simulink model "finalsimple_VER"  (R2023b)
settings: Solver=VariableStepAuto  StartTime=0.0  StopTime=5  FixedStep=4  MaxStep=0.01  RelTol=1e-3
undefined symbols (not defined in the file or in its folder): Ion, Lithium
libraries: simulink x40, nesl_utility x10, spsSeriesRLCBranchLib x8, fl_lib x6, spsMosfetLib x6, dspsrcs4 x5, spsControlledCurrentSourceLib x5, ee_lib x4, spsCurrentMeasurementLib x4, spsVoltageMeasurementLib x4, spsBatteryLib x3, spsGroundLib x2
(part 1 of 2)
settings Model: Creator=yeowy  LastModifiedBy=yeowy
settings DataIOCC: SaveFinalState=on  SaveOperatingPoint=on  SaveFormat=StructureWithTime

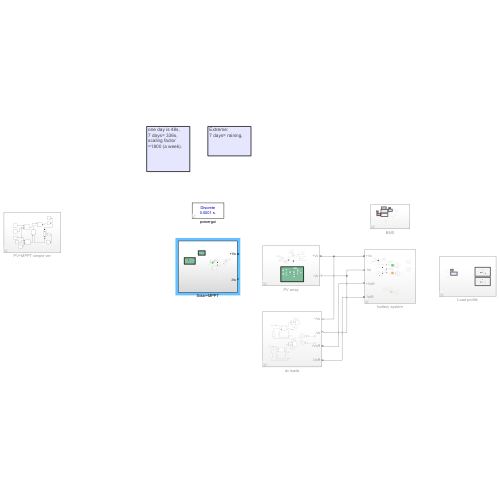
[thumbnail: Simulink's stored preview of the top-level diagram]
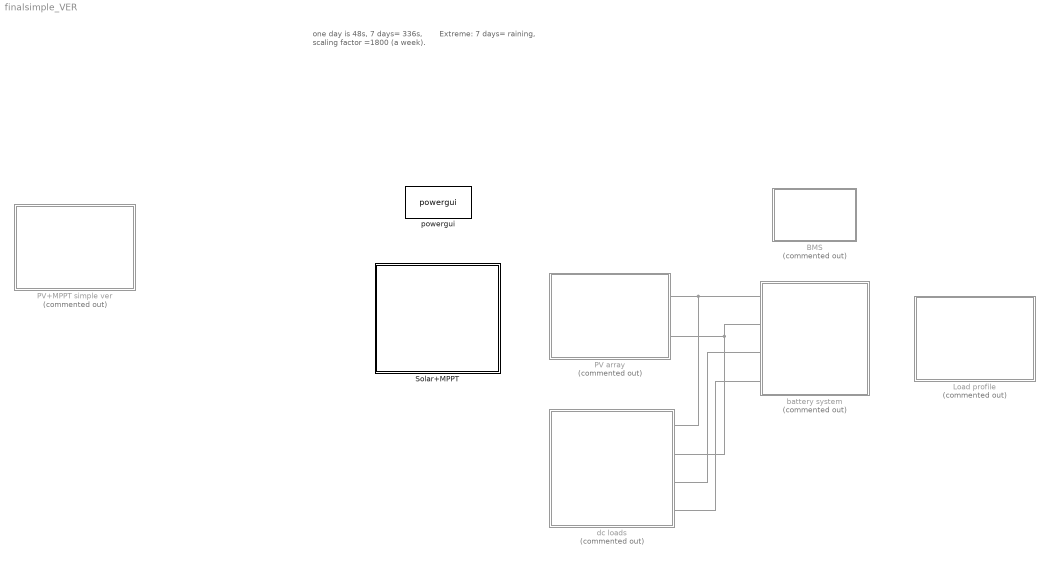
== system finalsimple_VER ==
  note: Extreme:
      | 7 days= raining,
  note: one day is 48s,
      | 7 days= 336s,
      | scaling factor
      | =1800 (a week).
  BMS : Subsystem  Commented=on
  Load profile : Subsystem  Commented=on
  PV array : Subsystem  Commented=on
  PV+MPPT simple ver : Subsystem  Commented=on
  Solar+MPPT : Subsystem
  battery system : Subsystem  Commented=on
  dc loads : Subsystem  Commented=on
  powergui : sps_lib/powergui  Priority=1  SimulationMode=Discrete  SampleTime=1e-4  frequency=60  Iterations=50  frequencyindice=0  Pbase=100e6  ErrMax=1e-4  UnitsV=kV  UnitsW=MW  buscounter=0  FunctionMessages=off  echomessages=off  EnableUseOfTLC=off  CurrentSourceSwitches=off  DisableSnubberDevices=off  DisableRonSwitches=off  DisableVfSwitches=off  DisplayEquations=off  AutomaticDiscreteSolvers=off  SolverType=Tustin/Backward Euler (TBE)  Interpol=off  ExternalGateDelay=off  methode=off  Ts=100  x0status=blocks  SPID=on  SwTol=0  HookPort=off  NonlinearTolerance=1e-4  nMaxIteration=100  ContinueOnMaxIteration=off  RestoreLinks=warning  ResistiveCurrentMeasurement=off  Frange=[0:2:500]  Ylog=off  Xlog=on  ShowGrid=off  save=off  variable=ZData  structure=0  ZoomFFT=off  StartTime=0.0  cycles=1  DisplayStyle=1  fundamental=60  FreqAxis=off  MaxFrequency=1000  frequencyindicesteady=1  RmsSteady=1  display=off
  connections:
  PV array/RConn1 -- dc loads/RConn1 -- battery system/LConn1
  battery system/LConn2 -- dc loads/RConn2 -- PV array/RConn2
  battery system/LConn3 -- dc loads/RConn3
  battery system/LConn4 -- dc loads/RConn4

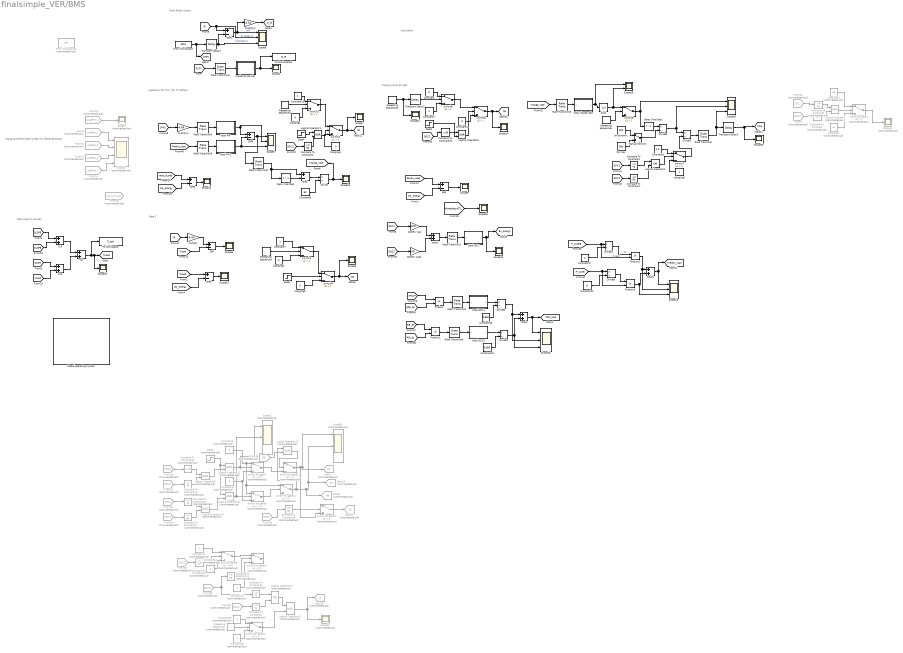
== system finalsimple_VER/BMS ==
  note: charging rover at night
  note: Calculation
  note: Total Load (in one day)
  note: Charging scheme:
      | 6pm to 6am for diesel generator
  note: Solar Panel system
  note: prediction (for tmr) (for PV battery)
  note: Gate 2
  Abs1 : Abs  SaturateOnIntegerOverflow=off
  Compare To Constant : simulink/Logic and Bit Operations/Compare To Constant  Commented=on  relop=<=  const=70  OutDataTypeStr=boolean
  Compare To Constant1 : simulink/Logic and Bit Operations/Compare To Constant  Commented=on  relop=>=  const=50  OutDataTypeStr=boolean
  Compare To Constant10 : simulink/Logic and Bit Operations/Compare To Constant  relop=>  const=85  OutDataTypeStr=boolean
  Compare To Constant11 : simulink/Logic and Bit Operations/Compare To Constant  Commented=on  relop=<=  const=20  OutDataTypeStr=boolean
  Compare To Constant12 : simulink/Logic and Bit Operations/Compare To Constant  Commented=on  relop=>  const=20  OutDataTypeStr=boolean
  Compare To Constant13 : simulink/Logic and Bit Operations/Compare To Constant  Commented=on  relop=<=  const=80  OutDataTypeStr=boolean
  Compare To Constant14 : simulink/Logic and Bit Operations/Compare To Constant  Commented=on  relop=<=  const=85  OutDataTypeStr=boolean
  Compare To Constant15 : simulink/Logic and Bit Operations/Compare To Constant  Commented=on  relop=>=  const=70  OutDataTypeStr=boolean
  Compare To Constant16 : simulink/Logic and Bit Operations/Compare To Constant  Commented=on  relop=<=  const=20  OutDataTypeStr=boolean
  Compare To Constant17 : simulink/Logic and Bit Operations/Compare To Constant  Commented=on  relop=<=  const=80  OutDataTypeStr=boolean
  Compare To Constant18 : simulink/Logic and Bit Operations/Compare To Constant  Commented=on  relop===  const=80  OutDataTypeStr=boolean
  Compare To Constant2 : simulink/Logic and Bit Operations/Compare To Constant  relop=>=  const=90  OutDataTypeStr=boolean
  Compare To Constant3 : simulink/Logic and Bit Operations/Compare To Constant  relop=>=  const=70  OutDataTypeStr=boolean
  Compare To Constant4 : simulink/Logic and Bit Operations/Compare To Constant  relop=<=  const=50  OutDataTypeStr=boolean
  Compare To Constant9 : simulink/Logic and Bit Operations/Compare To Constant  Commented=on  relop=<=  const=20  OutDataTypeStr=boolean
  Constant : Constant  Value=0
  Constant1 : Constant
  Constant{4,11,14,19} (4 alike) : Constant  Commented=on
  Constant12 : Constant  Commented=on  Value=0
  Constant13 : Constant
  Constant15 : Constant  Value=9.950
  Constant16 : Constant  Value=9.950
  Constant17 : Constant  Value=4
  Constant18 : Constant  Commented=on  Value=0
  Constant2 : Constant  Value=0
  Constant20 : Constant  Value=6
  Constant3 : Constant  Commented=on  Value=0
  Constant5 : Constant  Commented=on  Value=40
  Constant6 : Constant  Value=50
  Constant7 : Constant
  Constant8 : Constant  Value=1.3
  Constant9 : Constant  Commented=on  Value=80
  Delay One Step : Delay  DelayLength=1
  Delay One Step1 : Delay  DelayLength=1  SampleTime=50
  Diesel operating system : Subsystem
  Diff{,1..5} (6 alike) : Sum  Inputs=+-
  Divide{,1..6} (7 alike) : Product  Inputs=*/  RndMeth=Zero  SaturateOnIntegerOverflow=on
  From Workspace : FromWorkspace  VariableName=data  SampleTime=50  OutputAfterFinalValue=Holding final value
  From Workspace1 : FromWorkspace  Commented=on  VariableName=PIR
  From10 : From  Commented=on  GotoTag=LoadPre_3  TagVisibility=global
  From12 : From  Commented=on  GotoTag=LoadPre_4  TagVisibility=global
  From13 : From  Commented=on  GotoTag=LoadPre_1  TagVisibility=global
  From14 : From  Commented=on  GotoTag=LoadPre_7  TagVisibility=global
  From20 : From  Commented=on  GotoTag=Next_2hLoad  TagVisibility=global
  From23 : From  Commented=on  GotoTag=SOC1  TagVisibility=global
  From30 : From  Commented=on  GotoTag=SOC3  TagVisibility=global
  From{7,32,35..37} (5 alike) : From  Commented=on  GotoTag=SOC2  TagVisibility=global
  From33 : From  Commented=on  GotoTag=SOC3  TagVisibility=global
  From34 : From  Commented=on  GotoTag=SOC3
  From38 : From  Commented=on  GotoTag=SOC3
  From39 : From  Commented=on  GotoTag=G5  TagVisibility=global
  From5 : From  Commented=on  GotoTag=LoadPre_2  TagVisibility=global
  Goto13 : Goto  Commented=on  GotoTag=L1  TagVisibility=global
  Goto14 : Goto  Commented=on  GotoTag=G4  TagVisibility=global
  Goto15 : Goto  Commented=on  GotoTag=G5  TagVisibility=global
  Goto7 : Goto  Commented=on  GotoTag=G2  TagVisibility=global
  Goto8 : Goto  Commented=on  GotoTag=G6  TagVisibility=global
  Logical Operator{,8,10..12,16} (6 alike) : Logic  Commented=on  AllPortsSameDT=off  OutDataTypeStr=boolean
  Logical Operator1 : Logic  Operator=XOR  AllPortsSameDT=off  OutDataTypeStr=boolean
  Logical Operator13 : Logic  Commented=on  Operator=XOR  AllPortsSameDT=off  OutDataTypeStr=boolean
  Logical Operator15 : Logic  Commented=on  Operator=OR  AllPortsSameDT=off  OutDataTypeStr=boolean
  Logical Operator2 : Logic  Operator=OR  AllPortsSameDT=off  OutDataTypeStr=boolean
  Logical Operator9 : Logic  Operator=XOR  AllPortsSameDT=off  OutDataTypeStr=boolean
  Manual Switch2 : ManualSwitch
  Multiply : Gain  Gain=4.64
  Multiply1 : Gain  Gain=4.64
  Multiply2 : Gain  Gain=4.64
  Product{,1..3} (4 alike) : Product
  Rate Transition : RateTransition  OutPortSampleTime=600
  Rate Transition1 : RateTransition  OutPortSampleTime=100
  Rate Transition{2..3,6,8..9} (5 alike) : RateTransition  OutPortSampleTime=50
  Rate Transition4 : RateTransition  OutPortSampleTime=100
  Rate Transition5 : RateTransition  OutPortSampleTime=100
  Repeating Sequence1 : simulink/Sources/Repeating Sequence  Commented=on  rep_seq_t=[0 300 300.1 900.99 901 1200]  rep_seq_y=[0.9 0.9 1.01 1.01 0.9 0.9]
  Repeating Sequence2 : simulink/Sources/Repeating Sequence  rep_seq_t=[0 300 300.1 900.99 901 1200]  rep_seq_y=[0.9 0.9 1.01 1.01 0.9 0.9]
  Repeating Sequence3 : simulink/Sources/Repeating Sequence  rep_seq_t=[0 300 300.1 900.99 901 1200]  rep_seq_y=[0.9 0.9 1.01 1.01 0.9 0.9]
  Repeating Sequence4 : simulink/Sources/Repeating Sequence  rep_seq_t=[0 300 300.1 900.99 901 1200]  rep_seq_y=[0.9 0.9 1.01 1.01 0.9 0.9]
  Repeating Sequence5 : simulink/Sources/Repeating Sequence  rep_seq_t=[0 1099.99 1100 1200 1200.1]  rep_seq_y=[0.9 0.9 1.01 1.01 0.9]
  Scope{1,4,7..10,12..15,17,23..25} (14 alike) : Scope
  Scope11 : Scope  Commented=on
  Scope{5..6,16,19,26} (5 alike) : Scope  NumInputPorts=3
  Scope18 : Scope  NumInputPorts=2
  Scope2 : Scope  Commented=on  NumInputPorts=4
  Scope20 : Scope  Commented=on  NumInputPorts=3
  Scope21 : Scope  Commented=on  NumInputPorts=3
  Scope22 : Scope  Commented=on
  Scope3 : Scope  Commented=on
  Step1 : Step  Time=2400  After=2  SampleTime=1
  Step2 : Step  Time=2400  After=2  SampleTime=1
  Step3 : Step  Commented=on  Time=2400  After=2  SampleTime=1
  Step4 : Step  Time=2400  After=2  SampleTime=1
  TL5 : Sum
  TL6 : Sum
  TL7 : Sum
  To Workspace : ToWorkspace  VariableName=TLoad  SampleTime=1
      settings: Decimation=2  Save2DSignal=2-D array (concatenate along first dimension)
  To Workspace1 : ToWorkspace  VariableName=D_IR  SampleTime=1
      settings: Decimation=2  Save2DSignal=2-D array (concatenate along first dimension)
  Transport Delay1 : TransportDelay  DelayTime=2400
  Transport Delay2 : TransportDelay  DelayTime=2400
  Transport Delay3 : TransportDelay  DelayTime=900
  battery cap : Gain  Gain=100
  battery cap1 : Gain  Gain=50
  charging{1..4} (4 alike) : Constant  Value=0
  charging5 : Constant
  for dynamic : Constant  Value=300
  for max : Constant  Value=500
  gap : Sum  Inputs=+-
  irradiance per day : MATLAB Function  TreatAsAtomicUnit=on
  switch for gate{1,11..13} (4 alike) : Switch  Commented=on  Criteria=u2 > Threshold  SaturateOnIntegerOverflow=off  InputSameDT=off
  switch for gate{7..10} (4 alike) : Switch  Commented=on  Criteria=u2 ~= 0  Threshold=1  SaturateOnIntegerOverflow=off  InputSameDT=off
  switch for gate14 : Switch  Commented=on  Criteria=u2 > Threshold  Threshold=1  SaturateOnIntegerOverflow=off  InputSameDT=off
  switch{1,3..6,8} (6 alike) : Switch  Criteria=u2 > Threshold  Threshold=1  SaturateOnIntegerOverflow=off  InputSameDT=off
  switch2 : Switch  Criteria=u2 > Threshold  SaturateOnIntegerOverflow=off  InputSameDT=off
  switch7 : Switch  Criteria=u2 > Threshold  SaturateOnIntegerOverflow=off  InputSameDT=off
  total PIR : MATLAB Function  TreatAsAtomicUnit=on
  total PIR1 : MATLAB Function  TreatAsAtomicUnit=on
  total SOC : MATLAB Function  TreatAsAtomicUnit=on
  total SOC1 : MATLAB Function  TreatAsAtomicUnit=on
  total SOC2 : MATLAB Function  TreatAsAtomicUnit=on
  total charge rate : MATLAB Function  TreatAsAtomicUnit=on
  total1 : Sum
  total2 : Sum
  total3 : Sum
  tag scope: Bs_energy=global, CR4=global, D_IR=global, G1=global, G2=global, G4=global, Predict_load=global, TDC_load=global, TLoad=global, charge_rate=global
  wires:
  Diff/1 -> Scope4/1
  From Workspace/1 -> [PIR], Transport Delay1/1
  Diff1/1 -> Multiply2/1, Scope6/1  "Diff"
  From14/1 -> Scope2/4
  From12/1 -> Scope2/3
  From10/1 -> Scope2/2
  From5/1 -> Scope2/1
  From13/1 -> Scope3/1
  [IR] -> Multiply/1
  Multiply/1 -> Diff/1
  Multiply1/1 -> Rate Transition3/1
  [PIR] -> Multiply1/1
  Diff4/1 -> Rate Transition8/1, Scope5/1
  [IR] -> Diff1/1, Scope6/2  "Expected IR"
  [D_IR] -> Rate Transition2/1
  Rate Transition2/1 -> irradiance per day/1(u)
  irradiance per day/1(y) -> To Workspace1/1, Scope1/1
  Multiply2/1 -> [D_IR]
  [DLSPB] -> TL5/1
  [CLSPB] -> TL5/2
  [DLRB] -> TL6/1
  [CLRB] -> TL6/2
  TL6/1 -> TL7/2
  TL5/1 -> TL7/1
  TL7/1 -> To Workspace/1, Scope17/1, [TLoad]
  [TLoad] -> Diff/2
  [Bs_energy] -> Diff3/2
  [TLoad] -> Diff3/1
  Diff3/1 -> Scope13/1
  [Bs_energy] -> Diff5/2
  [Next_dLoad] -> Diff5/1
  Diff5/1 -> Scope14/1
  charging2/1 -> switch3/3
  Constant7/1 -> switch3/1
  Repeating Sequence2/1 -> Transport Delay2/1, Scope12/1
  Transport Delay2/1 -> switch5/2
  Constant/1 -> switch5/1
  Constant1/1 -> switch5/3
  switch5/1 -> switch6/1
  Step2/1 -> Logical Operator9/2
  [SOC2] -> Compare To Constant10/1
  Compare To Constant10/1 -> Logical Operator9/1
  Logical Operator9/1 -> switch6/2
  Constant2/1 -> switch6/3
  switch6/1 -> Scope24/1, [G4]
  From35/1 -> Compare To Constant12/1
  From30/1 -> Compare To Constant11/1
  Constant12/1 -> switch for gate9/3
  Compare To Constant11/1 -> switch for gate9/2
  Constant11/1 -> switch for gate9/1
  Compare To Constant14/1 -> switch for gate10/2
  Constant14/1 -> switch for gate10/3
  From33/1 -> Compare To Constant14/1, Compare To Constant15/1
  switch for gate9/1 -> switch for gate10/1
  From36/1 -> Compare To Constant9/1
  Constant19/1 -> switch for gate14/3
  Constant18/1 -> switch for gate14/1
  Repeating Sequence1/1 -> switch for gate14/2
  Compare To Constant15/1 -> Logical Operator15/1
  Compare To Constant9/1 -> Logical Operator15/2
  Logical Operator15/1 -> Logical Operator16/1
  switch for gate14/1 -> Logical Operator16/2
  Logical Operator16/1 -> Scope22/1, Goto13/1
  From32/1 -> Compare To Constant13/1
  Compare To Constant12/1 -> Logical Operator8/1
  Compare To Constant13/1 -> Logical Operator8/2
  Step3/1 -> Logical Operator11/1, Logical Operator12/1
  Logical Operator8/1 -> Logical Operator12/2
  Logical Operator12/1 -> Scope21/1, switch for gate7/2
  switch for gate7/1 -> switch for gate12/3
  Constant3/1 -> switch for gate8/3, switch for gate7/3
  Constant4/1 -> switch for gate11/1, switch for gate8/1, switch for gate7/1
  Compare To Constant17/1 -> Logical Operator10/2
  Compare To Constant16/1 -> Logical Operator10/1
  From34/1 -> Compare To Constant17/1
  Logical Operator10/1 -> Logical Operator11/2
  Logical Operator11/1 -> Scope21/2, switch for gate8/2
  switch for gate11/1 -> Logical Operator13/1, Goto8/1, Scope20/2, Goto14/1
  From38/1 -> Compare To Constant18/1
  Compare To Constant18/1 -> switch for gate13/2
  switch for gate13/1 -> Goto15/1
  switch for gate8/1 -> switch for gate11/2
  From37/1 -> Compare To Constant16/1
  switch for gate12/1 -> switch for gate13/3, Goto7/1, Scope20/1
  From39/1 -> Logical Operator13/2
  Logical Operator13/1 -> switch for gate12/2
  Transport Delay1/1 -> Diff1/2, Scope6/3  "Predicted IR"
  [SOC2] -> battery cap1/1
  [SOC1] -> battery cap/1
  battery cap1/1 -> total1/2
  battery cap/1 -> total1/1
  [Seven_Load] -> gap/1
  [Bs_energy] -> gap/2
  gap/1 -> Scope9/1
  total1/1 -> Rate Transition1/1
  total SOC/1(y) -> Scope10/1, [Bs_energy]
  Constant9/1 -> switch for gate1/1
  Constant5/1 -> switch for gate1/3
  switch for gate1/1 -> Scope11/1
  From7/1 -> Compare To Constant/1
  Compare To Constant/1 -> Logical Operator/2
  Compare To Constant1/1 -> Logical Operator/1
  From23/1 -> Compare To Constant1/1
  Logical Operator/1 -> switch for gate1/2
  Rate Transition1/1 -> total SOC/1(u)
  Repeating Sequence3/1 -> switch3/2
  Rate Transition3/1 -> total PIR/1(u)
  total PIR/1(y) -> Diff4/1, Scope5/2
  [threedaysTL] -> Scope15/1
  [RB_Sp] -> Product1/2
  [SPB_ET] -> Product/1
  [RB_ET] -> Product1/1
  [SPB_Sp] -> Product/2
  Rate Transition4/1 -> total SOC1/1(u)
  Product/1 -> Rate Transition4/1
  Rate Transition5/1 -> total SOC2/1(u)
  Product1/1 -> Rate Transition5/1
  total2/1 -> Scope16/1, [TDC_load]
  [Predict_load] -> Rate Transition9/1
  Delay One Step/1 -> Diff2/2
  Diff2/1 -> Divide/1
  Constant6/1 -> Divide/2
  Divide/1 -> [charge_rate], Scope23/1
  Rate Transition6/1 -> total charge rate/1(u)
  [charge_rate] -> Rate Transition6/1
  Step1/1 -> switch4/2
  charging3/1 -> switch4/3
  switch3/1 -> switch4/1
  switch4/1 -> Scope8/1, [G2]
  switch2/1 -> [G1], Scope7/1
  switch1/1 -> switch2/1
  charging4/1 -> switch2/3
  Repeating Sequence4/1 -> switch1/2
  Constant13/1 -> switch1/1
  charging1/1 -> switch1/3
  total SOC1/1(y) -> Divide2/1
  Divide2/1 -> Scope16/2, total2/1
  total SOC2/1(y) -> Divide3/1
  Constant15/1 -> Divide2/2
  Constant16/1 -> Divide3/2
  Divide3/1 -> total2/2, Scope16/3
  Constant17/1 -> Divide4/2
  [P_CLSPB] -> Product2/2, Divide4/1  "Speed"
  Divide4/1 -> Product2/1  "Te"
  Divide5/1 -> Product3/1
  Constant20/1 -> Divide5/2
  [P_CLRB] -> Product3/2, Divide5/1
  Product2/1 -> Scope19/2, total3/1
  Product3/1 -> Scope19/3, total3/2
  total3/1 -> Scope19/1, [Predict_load]
  total charge rate/1(y) -> Scope18/1, Abs1/1
  Divide1/1 -> Rate Transition/1
  Repeating Sequence5/1 -> switch8/2
  Abs1/1 -> Scope18/2, switch8/1
  Transport Delay3/1 -> Scope25/1, [CR4]
  Rate Transition8/1 -> Delay One Step/1, Diff2/1
  [SOC1] -> Compare To Constant2/1
  Logical Operator1/1 -> switch2/2
  Compare To Constant2/1 -> Logical Operator1/2
  Step4/1 -> Logical Operator1/1
  for dynamic/1 -> Manual Switch2/1
  for max/1 -> Manual Switch2/2
  Rate Transition9/1 -> total PIR1/1(u)
  total PIR1/1(y) -> Scope5/3, Diff4/2
  Manual Switch2/1 -> Divide6/2
  Divide6/1 -> Divide1/1, Scope26/2
  charging5/1 -> switch7/3
  Constant8/1 -> switch7/1
  [SOC2] -> Compare To Constant3/1
  switch7/1 -> Divide1/2
  Compare To Constant3/1 -> Logical Operator2/1
  [SOC1] -> Compare To Constant4/1
  Logical Operator2/1 -> switch7/2
  Compare To Constant4/1 -> Logical Operator2/2
  switch8/1 -> Delay One Step1/1, Scope26/1
  Rate Transition/1 -> Transport Delay3/1, Scope26/3
  Delay One Step1/1 -> Divide6/1

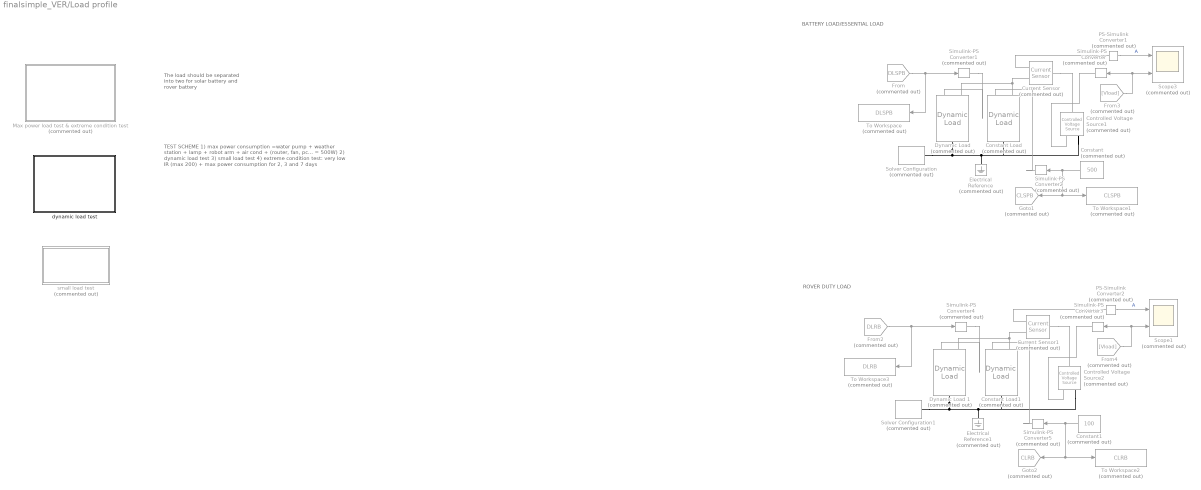
== system finalsimple_VER/Load profile ==
  note: ROVER DUTY LOAD
  note: BATTERY LOAD/ESSENTIAL LOAD
  note: The load should be
      | separated into two
      | for solar battery
      | and rover battery
  note: TEST SCHEME
      | 1) max power consumption
      | =water pump + weather station + lamp
      |  + robot arm + air cond + (router, fan, pc... = 500W)
      | 2) dynamic load test
      | 3) small load test
      | 4) extreme condition test:
      | very low IR (max 200) + max power consumption
      | for 2, 3 and 7 days
  Constant : Constant  Commented=on  Value=500
  Constant Load : ee_lib/Passive/Dynamic Load  Commented=on  load_type=ee.enum.dc_ac.dc  min_supply_voltage=45 V  pow_min=1 W  G_reverse=1e-6 S  deltaV=1e-3 V  f0=60 Hz  Vrms_min=200 V  Pmin=1e-3 W  enable_fault=simscape.enum.onoff.off  fault_action=simscape.enum.assert.action.none  t_fault=1 s  open_conductance=1e-4 S
      settings: InternalSimscapePortConfiguration="{\"Bottom\":[],\"Left\":[{\"id\":\"p\",\"label\":\"+\",\"type\":\"foundation.electrical.electrical\"}],\"Right\":[{\"id\":\"n\",\"label\":\"-\",\"type\":\"foundation.electrical.electrical\"}],\"Top\":[{\"id\":\"P\",\"label\":\"P\",\"type\":\"input\"}]}"
  Constant Load1 : ee_lib/Passive/Dynamic Load  Commented=on  load_type=ee.enum.dc_ac.dc  min_supply_voltage=45 V  pow_min=1 W  G_reverse=1e-6 S  deltaV=1e-3 V  f0=60 Hz  Vrms_min=200 V  Pmin=1e-3 W  enable_fault=simscape.enum.onoff.off  fault_action=simscape.enum.assert.action.none  t_fault=1 s  open_conductance=1e-4 S
      settings: InternalSimscapePortConfiguration="{\"Bottom\":[],\"Left\":[{\"id\":\"p\",\"label\":\"+\",\"type\":\"foundation.electrical.electrical\"}],\"Right\":[{\"id\":\"n\",\"label\":\"-\",\"type\":\"foundation.electrical.electrical\"}],\"Top\":[{\"id\":\"P\",\"label\":\"P\",\"type\":\"input\"}]}"
  Constant1 : Constant  Commented=on  Value=100
  Controlled Voltage Source1 : fl_lib/Electrical/Electrical Sources/Controlled Voltage Source  Commented=on
  Controlled Voltage Source2 : fl_lib/Electrical/Electrical Sources/Controlled Voltage Source  Commented=on
  Current Sensor : fl_lib/Electrical/Electrical Sensors/Current Sensor  Commented=on
  Current Sensor1 : fl_lib/Electrical/Electrical Sensors/Current Sensor  Commented=on
  "Dynamic Load " : ee_lib/Passive/Dynamic Load  Commented=on  load_type=ee.enum.dc_ac.dc  min_supply_voltage=45 V  pow_min=1 W  G_reverse=1e-6 S  deltaV=1e-3 V  f0=60 Hz  Vrms_min=200 V  Pmin=1e-3 W  enable_fault=simscape.enum.onoff.off  fault_action=simscape.enum.assert.action.none  t_fault=1 s  open_conductance=1e-4 S
      settings: InternalSimscapePortConfiguration="{\"Bottom\":[],\"Left\":[{\"id\":\"p\",\"label\":\"+\",\"type\":\"foundation.electrical.electrical\"}],\"Right\":[{\"id\":\"n\",\"label\":\"-\",\"type\":\"foundation.electrical.electrical\"}],\"Top\":[{\"id\":\"P\",\"label\":\"P\",\"type\":\"input\"}]}"
  Dynamic Load 1 : ee_lib/Passive/Dynamic Load  Commented=on  load_type=ee.enum.dc_ac.dc  min_supply_voltage=45 V  pow_min=1 W  G_reverse=1e-6 S  deltaV=1e-3 V  f0=60 Hz  Vrms_min=200 V  Pmin=1e-3 W  enable_fault=simscape.enum.onoff.off  fault_action=simscape.enum.assert.action.none  t_fault=1 s  open_conductance=1e-4 S
      settings: InternalSimscapePortConfiguration="{\"Bottom\":[],\"Left\":[{\"id\":\"p\",\"label\":\"+\",\"type\":\"foundation.electrical.electrical\"}],\"Right\":[{\"id\":\"n\",\"label\":\"-\",\"type\":\"foundation.electrical.electrical\"}],\"Top\":[{\"id\":\"P\",\"label\":\"P\",\"type\":\"input\"}]}"
  Electrical Reference : fl_lib/Electrical/Electrical Elements/Electrical Reference  Commented=on
  Electrical Reference1 : fl_lib/Electrical/Electrical Elements/Electrical Reference  Commented=on
  From : From  Commented=on  GotoTag=DLSPB  TagVisibility=global
  From2 : From  Commented=on  GotoTag=DLRB  TagVisibility=global
  From3 : From  Commented=on  GotoTag=Vload
  From4 : From  Commented=on  GotoTag=Vload
  Goto1 : Goto  Commented=on  GotoTag=CLSPB  TagVisibility=global
  Goto2 : Goto  Commented=on  GotoTag=CLRB  TagVisibility=global
  Max power load test & extreme condition test : Subsystem  Commented=on
  PS-Simulink Converter1 : nesl_utility/PS-Simulink Converter  Commented=on  PhysicalDomain=network_engine_domain  SubClassName=ps_output  LeftPortType=input  RightPortType=output  PseudoPeriodic=off  Frequencies=[]  VectorFormat=inherit  Unit=inherit  AffineConversion=off
  PS-Simulink Converter2 : nesl_utility/PS-Simulink Converter  Commented=on  PhysicalDomain=network_engine_domain  SubClassName=ps_output  LeftPortType=input  RightPortType=output  PseudoPeriodic=off  Frequencies=[]  VectorFormat=inherit  Unit=inherit  AffineConversion=off
  Scope1 : Scope  Commented=on  NumInputPorts=2
  Scope3 : Scope  Commented=on  NumInputPorts=2
  Simulink-PS Converter{,1..5} (6 alike) : nesl_utility/Simulink-PS Converter  Commented=on  PhysicalDomain=network_engine_domain  SubClassName=ps_input  LeftPortType=input  RightPortType=output  PseudoPeriodic=off  Frequencies=[]  NoiseDistribution=none  NoiseParameters=[]  Unit=1  AffineConversion=off  FilteringAndDerivatives=provide  SimscapeFilterOrder=1  InputFilterTimeConstant=0.001  UdotUserProvided=0
  Solver Configuration : nesl_utility/Solver Configuration  Commented=on  PhysicalDomain=network_engine_domain  SubClassName=solver  LeftPortType=input  RightPortType=generic  Tones=[]  Harmonics=[]  SimulateNoise=off  Profile=off  UseLocalSampling=off  EnableSwitchedLinearOptims=on  FrequencyDomain=off  UseCCode=off  RelTol=0.001  AbsTol=0.001  MinStep=1e-09  ToWorkspace=off  RevertToSquareIcSolve=off  NumHomotopyIterations=100  PhasorMode=off  PhasorModeNumHarmonics=1  ConsistencySolver=NEWTON_XTOL_AFTER_FTOL  IndexReductionMethod=DerivativeReplacement  DoDC=off  ResidualTolerance=1e-09  ConsistencyTolSource=GLOBAL  ConsistencyAbsTol=0.001  ConsistencyRelTol=0.001  ConsistencyTolFactor=0.001  UseLocalSolver=off  LocalSolverChoice=NE_BACKWARD_EULER_ADVANCER  ResolveIndetEquations=on  FunctionEvalNumThread=1  LocalSolverSampleTime=0.001  DoFixedCost=off  MaxNonlinIter=3  MaxModeIter=2  ComputeImpulses=off  ImpulseIterations=2  LinearAlgebra=auto  LinearAlgebraNumThread=0  EquationFormulation=NE_TIME_EF  DelaysMemoryBudget=1024  AutomaticFiltering=on  FilteringTimeConstant=0.001  PartitionStorageMethod=AS_NEEDED  PartitionMemoryBudget=1024  PartitionMethod=ROBUST  MultibodyUseLocalSolver=off  MultibodyLocalSolverChoice=ODE1  MultibodyLocalSolverSampleTime=0.001
  Solver Configuration1 : nesl_utility/Solver Configuration  Commented=on  PhysicalDomain=network_engine_domain  SubClassName=solver  LeftPortType=input  RightPortType=generic  Tones=[]  Harmonics=[]  SimulateNoise=off  Profile=off  UseLocalSampling=off  EnableSwitchedLinearOptims=on  FrequencyDomain=off  UseCCode=off  RelTol=0.001  AbsTol=0.001  MinStep=1e-09  ToWorkspace=off  RevertToSquareIcSolve=off  NumHomotopyIterations=100  PhasorMode=off  PhasorModeNumHarmonics=1  ConsistencySolver=NEWTON_XTOL_AFTER_FTOL  IndexReductionMethod=DerivativeReplacement  DoDC=off  ResidualTolerance=1e-09  ConsistencyTolSource=GLOBAL  ConsistencyAbsTol=0.001  ConsistencyRelTol=0.001  ConsistencyTolFactor=0.001  UseLocalSolver=off  LocalSolverChoice=NE_BACKWARD_EULER_ADVANCER  ResolveIndetEquations=on  FunctionEvalNumThread=1  LocalSolverSampleTime=0.001  DoFixedCost=off  MaxNonlinIter=3  MaxModeIter=2  ComputeImpulses=off  ImpulseIterations=2  LinearAlgebra=auto  LinearAlgebraNumThread=0  EquationFormulation=NE_TIME_EF  DelaysMemoryBudget=1024  AutomaticFiltering=on  FilteringTimeConstant=0.001  PartitionStorageMethod=AS_NEEDED  PartitionMemoryBudget=1024  PartitionMethod=ROBUST  MultibodyUseLocalSolver=off  MultibodyLocalSolverChoice=ODE1  MultibodyLocalSolverSampleTime=0.001
  To Workspace : ToWorkspace  Commented=on  VariableName=DLSPB  SaveFormat=Structure With Time  SampleTime=1
      settings: Decimation=2  Save2DSignal=2-D array (concatenate along first dimension)
  To Workspace1 : ToWorkspace  Commented=on  VariableName=CLSPB  SaveFormat=Structure With Time  SampleTime=1
      settings: Decimation=2  Save2DSignal=2-D array (concatenate along first dimension)
  To Workspace2 : ToWorkspace  Commented=on  VariableName=CLRB  SaveFormat=Structure With Time  SampleTime=1
      settings: Decimation=2  Save2DSignal=2-D array (concatenate along first dimension)
  To Workspace3 : ToWorkspace  Commented=on  VariableName=DLRB  SaveFormat=Structure With Time  SampleTime=1
      settings: Decimation=2  Save2DSignal=2-D array (concatenate along first dimension)
  dynamic load test : Subsystem
  small load test : Subsystem  Commented=on
  wires:
  From3/1 -> Scope3/2, Simulink-PS Converter/1
  PS-Simulink Converter1/1 -> Scope3/1  "A"
  Constant/1 -> To Workspace1/1, Goto1/1, Simulink-PS Converter2/1
  Constant1/1 -> Simulink-PS Converter5/1, To Workspace2/1, Goto2/1
  PS-Simulink Converter2/1 -> Scope1/1  "A"
  From4/1 -> Scope1/2, Simulink-PS Converter3/1
  From2/1 -> To Workspace3/1, Simulink-PS Converter4/1
  From/1 -> To Workspace/1, Simulink-PS Converter1/1
  connections:
  "Dynamic Load "/LConn1 -- Current Sensor/RConn2 -- Constant Load/LConn1
  "Dynamic Load "/RConn1 -- Electrical Reference/LConn1 -- Constant Load/RConn1 -- Controlled Voltage Source1/RConn2 -- Solver Configuration/RConn1
  Current Sensor/RConn1 -- PS-Simulink Converter1/LConn1
  Simulink-PS Converter1/RConn1 -- "Dynamic Load "/LConn2
  Current Sensor/LConn1 -- Controlled Voltage Source1/LConn1
  Simulink-PS Converter/RConn1 -- Controlled Voltage Source1/RConn1
  Simulink-PS Converter2/RConn1 -- Constant Load/LConn2
  Dynamic Load 1/LConn1 -- Current Sensor1/RConn2 -- Constant Load1/LConn1
  Dynamic Load 1/RConn1 -- Solver Configuration1/RConn1 -- Controlled Voltage Source2/RConn2 -- Constant Load1/RConn1 -- Electrical Reference1/LConn1
  Simulink-PS Converter5/RConn1 -- Constant Load1/LConn2
  Simulink-PS Converter3/RConn1 -- Controlled Voltage Source2/RConn1
  Current Sensor1/LConn1 -- Controlled Voltage Source2/LConn1
  Current Sensor1/RConn1 -- PS-Simulink Converter2/LConn1
  Simulink-PS Converter4/RConn1 -- Dynamic Load 1/LConn2

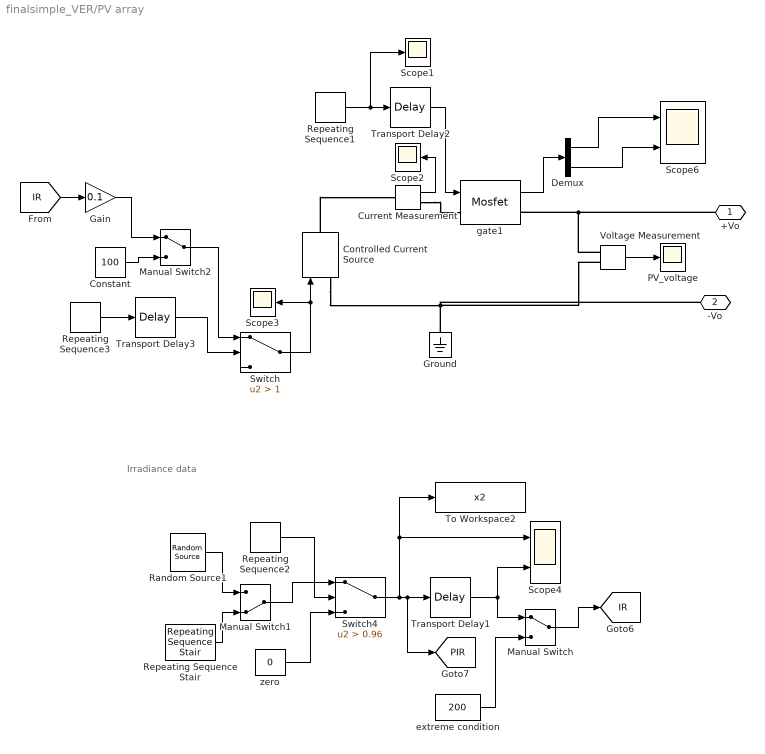
== system finalsimple_VER/PV array ==
  note: Irradiance data
  Constant : Constant  Value=100
  Controlled Current Source : spsControlledCurrentSourceLib/Controlled Current Source  Initialize=off  Source_Type=DC  Amplitude=160  Phase=0  Frequency=0  Measurements=Current
  Current Measurement : spsCurrentMeasurementLib/Current Measurement  PhasorSimulation=off  OutputType=Complex  PSBequivalent=0
  Demux : Demux  Outputs=2
  Gain : Gain  Gain=0.1
  Ground : spsGroundLib/Ground  LConnTagsString=a
  Manual Switch : ManualSwitch
  Manual Switch1 : ManualSwitch  CurrentSetting=0
  Manual Switch2 : ManualSwitch
  PV_voltage : Scope
  Random Source1 : dspsrcs4/Random Source  SrcType=Uniform  NormMethod=Ziggurat  CltLength=12  MinVal=200  MaxVal=1000  MeanVal=0  VarVal=1  RepMode=Not repeatable  rawSeed=1  IsInherit=off  SampMode=Discrete  SampTime=50  SampFrame=1  DataType=Double  OutComplex=Real  OutputFrames=off
  Repeating Sequence Stair : simulink/Sources/Repeating Sequence Stair  OutValues=[0 0 0 0 0 0 0 1 3 5 7 9 10 10 10 8 6 4 2 1 0 0 0 0].'*100  tsamp=50  OutMin=[]  OutMax=[]  OutDataTypeStr=double  OutputDataTypeScalingMode=double  OutDataType=fixdt(0,8)  ConRadixGroup=Best Precision: Vector-wise  OutScaling=2^-12
  Repeating Sequence1 : simulink/Sources/Repeating Sequence  rep_seq_t=[0 300 300.1 900.99 901 1200]  rep_seq_y=[0.9 0.9 1.01 1.01 0.9 0.9]
  Repeating Sequence2 : simulink/Sources/Repeating Sequence  rep_seq_t=[0 300 300.1 900.99 901 1200]  rep_seq_y=[0.9 0.9 1.01 1.01 0.9 0.9]
  Repeating Sequence3 : simulink/Sources/Repeating Sequence  rep_seq_t=[0 300 300.1 900.99 901 1200]  rep_seq_y=[0.9 0.9 1.01 1.01 0.9 0.9]
  Scope1 : Scope
  Scope2 : Scope
  Scope3 : Scope
  Scope4 : Scope  NumInputPorts=2
  Scope6 : Scope  NumInputPorts=2
  Switch : Switch  Criteria=u2 > Threshold  Threshold=1  SaturateOnIntegerOverflow=off  InputSameDT=off
  Switch4 : Switch  Criteria=u2 > Threshold  Threshold=0.96  RndMeth=Ceiling  ZeroCross=off  SaturateOnIntegerOverflow=off
  To Workspace2 : ToWorkspace  VariableName=x2  SaveFormat=Structure With Time  SampleTime=1
      settings: Decimation=2  Save2DSignal=2-D array (concatenate along first dimension)
  Transport Delay1 : TransportDelay  DelayTime=2400
  Transport Delay2 : TransportDelay  DelayTime=2400
  Transport Delay3 : TransportDelay  DelayTime=2400
  Voltage Measurement : spsVoltageMeasurementLib/Voltage Measurement  PhasorSimulation=off  OutputType=Complex  PSBequivalent=0
  extreme condition : Constant  Value=200
  gate1 : spsMosfetLib/Mosfet  Ron=0.1  Lon=0  Rd=0.1  Vfd=80  IC=0  Rs=1e5  Cs=inf  Measurements=on
  zero : Constant  Value=0  SampleTime=0
  +Vo : PMIOPort  Side=Right
  -Vo : PMIOPort  Port=2  Side=Right
  tag scope: IR=global, PIR=global
  wires:
  Switch/1 -> Controlled Current Source/1, Scope3/1
  Transport Delay3/1 -> Switch/2
  Repeating Sequence3/1 -> Transport Delay3/1
  Current Measurement/1 -> Scope2/1
  Transport Delay2/1 -> gate1/1
  Repeating Sequence1/1 -> Scope1/1, Transport Delay2/1
  gate1/1 -> Demux/1
  Demux/1 -> Scope6/1
  Demux/2 -> Scope6/2
  Constant/1 -> Manual Switch2/2
  [IR] -> Gain/1
  Manual Switch2/1 -> Switch/1
  Gain/1 -> Manual Switch2/1
  Voltage Measurement/1 -> PV_voltage/1
  Random Source1/1 -> Manual Switch1/1
  Manual Switch1/1 -> Switch4/1
  Switch4/1 -> To Workspace2/1, Scope4/1, Transport Delay1/1, [PIR]
  Repeating Sequence2/1 -> Switch4/2
  Manual Switch/1 -> [IR]
  Repeating Sequence Stair/1 -> Manual Switch1/2
  extreme condition/1 -> Manual Switch/2
  Transport Delay1/1 -> Scope4/2, Manual Switch/1
  zero/1 -> Switch4/3
  connections:
  Controlled Current Source/RConn1 -- Current Measurement/LConn1
  Controlled Current Source/LConn1 -- Voltage Measurement/LConn2 -- -Vo/RConn1 -- Ground/LConn1
  Current Measurement/RConn1 -- gate1/LConn1
  +Vo/RConn1 -- Voltage Measurement/LConn1 -- gate1/RConn1

== system finalsimple_VER/PV+MPPT simple ver ==
  Constant : Constant  Value=50
  Constant1 : Constant  Value=100
  Constant2 : Constant  Value=0
  Constant3 : Constant  Value=0
  Controlled Current Source : spsControlledCurrentSourceLib/Controlled Current Source  Initialize=on  Source_Type=AC  Amplitude=0  Phase=0  Frequency=0  Measurements=None
  Controlled Voltage Source : spsControlledVoltageSourceLib/Controlled Voltage Source  Initialize=on  Source_Type=DC  Amplitude=0  Phase=0  Frequency=0  Measurements=None
  Current Measurement1 : spsCurrentMeasurementLib/Current Measurement  PhasorSimulation=off  OutputType=Complex  PSBequivalent=0
  Repeating Sequence2 : simulink/Sources/Repeating Sequence  rep_seq_t=[0 11.99 12 35.99 36 48]  rep_seq_y=[0.9 0.9 1.01 1.01 0.9 0.9]
  Scope2 : Scope
  Scope3 : Scope
  Series RLC Branch2 : spsSeriesRLCBranchLib/Series RLC Branch  LConnTagsString=__new0  RConnTagsString=__new0  BranchType=R  Resistance=1  Inductance=1e-3  SetiL0=off  InitialCurrent=0  Capacitance=1e-6  Setx0=off  InitialVoltage=0  Measurements=None
  Switch1 : Switch  Criteria=u2 > Threshold  Threshold=0.96  RndMeth=Ceiling  ZeroCross=off  SaturateOnIntegerOverflow=off
  Switch2 : Switch  Criteria=u2 > Threshold  Threshold=0.96  RndMeth=Ceiling  ZeroCross=off  SaturateOnIntegerOverflow=off
  Voltage Measurement1 : spsVoltageMeasurementLib/Voltage Measurement  PhasorSimulation=off  OutputType=Complex  PSBequivalent=0
  wires:
  Constant1/1 -> Switch2/1
  Switch2/1 -> Controlled Current Source/1
  Constant2/1 -> Switch1/3
  Current Measurement1/1 -> Scope2/1
  Repeating Sequence2/1 -> Switch2/2, Switch1/2
  Voltage Measurement1/1 -> Scope3/1
  Constant3/1 -> Switch2/3
  Switch1/1 -> Controlled Voltage Source/1
  Constant/1 -> Switch1/1
  connections:
  Current Measurement1/RConn1 -- Voltage Measurement1/LConn1 -- Series RLC Branch2/LConn1
  Series RLC Branch2/RConn1 -- Controlled Voltage Source/LConn1 -- Voltage Measurement1/LConn2
  Controlled Current Source/LConn1 -- Controlled Voltage Source/RConn1
  Controlled Current Source/RConn1 -- Current Measurement1/LConn1

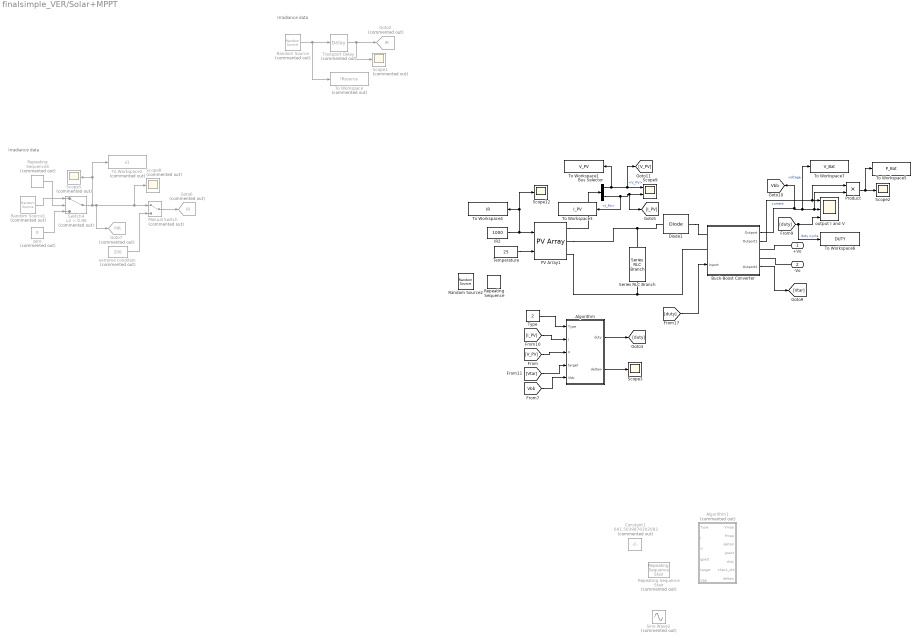
== system finalsimple_VER/Solar+MPPT ==
  note: Irradiance data
  note: Irradiance data
  Algorithm : MATLAB Function  TreatAsAtomicUnit=on
  Algorithm1 : MATLAB Function  Commented=on  TreatAsAtomicUnit=on
  Buck-Boost Converter : Subsystem
      settings: PortSchema="{\"entries\":[{\"content\":{\"sides\":[{\"content\":{\"connectorIds\":[\"LConn1\",\"LConn2\",\"In1\"]},\"type\":\"ConnectorPlacement.EquallySpacedRectSide\",\"uuid\":\"434e697c-d5be-45e6-bdc1-8ae755998e80\"},{\"content\":{\"connectorIds\":[\"Out1\",\"Out2\",\"RConn1\",\"RConn2\",\"Out3\"],\"side\":\"RIGHT\"},\"type\":\"ConnectorPlacement.EquallySpacedRectSide\",\"uuid\":\"10395034-5ec3-4cb8-9f4e-a5ff74166f8a\"},{\"content\":{\"side\":\"TOP\"},\"type\":\"ConnectorPlacement.EquallySpacedRectSide\",\"uuid\":\"7465b0d6-f669-4ab3-bc57-21c5b1d9d369\"}]},\"type\":\"ConnectorPlacement.EquallySpacedConnector\",\"uuid\":\"ddac4feb-4ed3-480d-95df-f0f80e961ae6\"}],\"packageUris\":[\"http://schema.mathworks.com/mf0/Connector/R2020b\"],\"version\":\"1.0\"}"
  Bus Selector : BusSelector  OutputSignals=V_PV,I_PV
  Constant1 : Constant  Commented=on  Value=601.5039876302083
  Diode1 : spsDiodeLib/Diode  Ron=0.001  Lon=0  Vf=0.8  IC=0  UseSnubber=0  Rs=500  Cs=250e-9  Measurements=off
  Goto2 : Goto  Commented=on  GotoTag=IR  TagVisibility=global
  Goto6 : Goto  Commented=on  GotoTag=IR  TagVisibility=global
  Goto7 : Goto  Commented=on  GotoTag=PIR  TagVisibility=global
  IR2 : Constant  Value=1000
  Manual Switch : ManualSwitch  Commented=on
  PV Array1 : spsPVArrayLib/PV Array  Npar=4  Nser=2  PlotType=array @ 25 deg.C & specified irradiances  S_vec="[ 1000  500  100 ]"  Temp_C_vec="[ 45 25  ]"  ModuleName=User-defined  PlotWhenSelected=off  Pm=580.0124  Ncell=144  Voc=51.4  Isc=14.22  Vm=43.22  Im=13.42  beta_Voc_pc=-0.36099  alpha_Isc_pc=0.102  beta_Voc=-0.18555  alpha_Isc=0.014504  IL=14.2363  I0=5.2538e-10  nI=0.5786  Rsh=331.4965  Rs=0.12745  RobustModel=off  RobustCellTemperature=313.3991  BAL=on  Tc=1e-6  Tfilter=5e-5
  Product : Product
  Random Source : dspsrcs4/Random Source  Commented=on  SrcType=Uniform  NormMethod=Ziggurat  CltLength=12  MinVal=200  MaxVal=1000  MeanVal=0  VarVal=1  RepMode=Not repeatable  rawSeed=1  IsInherit=off  SampMode=Discrete  SampTime=2  SampFrame=1  DataType=Double  OutComplex=Real  OutputFrames=off
  Random Source1 : dspsrcs4/Random Source  Commented=on  SrcType=Uniform  NormMethod=Ziggurat  CltLength=12  MinVal=200  MaxVal=1000  MeanVal=0  VarVal=1  RepMode=Not repeatable  rawSeed=1  IsInherit=off  SampMode=Discrete  SampTime=2  SampFrame=1  DataType=Double  OutComplex=Real  OutputFrames=off
  Random Source2 : dspsrcs4/Random Source  SrcType=Uniform  NormMethod=Ziggurat  CltLength=12  MinVal=500  MaxVal=1000  MeanVal=0  VarVal=1  RepMode=Not repeatable  rawSeed=1  IsInherit=off  SampMode=Discrete  SampTime=0.2  SampFrame=1  DataType=Double  OutComplex=Real  OutputFrames=off
  Repeating Sequence : simulink/Sources/Repeating Sequence  rep_seq_t=[0 2]  rep_seq_y=[200 1000]
  Repeating Sequence Stair : simulink/Sources/Repeating Sequence Stair  Commented=on  OutValues=[0 0 0 0 0 0 0 1 3 5 7 9 10 10 10 8 6 4 2 1 0 0 0 0].'*100  tsamp=2  OutMin=[]  OutMax=[]  OutDataTypeStr=double  OutputDataTypeScalingMode=double  OutDataType=fixdt(0,8)  ConRadixGroup=Best Precision: Vector-wise  OutScaling=2^-12
  Repeating Sequence4 : simulink/Sources/Repeating Sequence  Commented=on  rep_seq_t=[0 11.98 12 35.99 36 48]  rep_seq_y=[0.9 0.9 1.01 1.01 0.9 0.9]
  Scope1 : Scope  Commented=on
  Scope12 : Scope
  Scope2 : Scope
  Scope3 : Scope
  Scope5 : Scope  Commented=on
  Scope8 : Scope  Commented=on
  Scope9 : Scope  NumInputPorts=2
  Series RLC Branch : spsSeriesRLCBranchLib/Series RLC Branch  LConnTagsString=__new0  RConnTagsString=__new0  BranchType=C  Resistance=2  Inductance=1e-3  SetiL0=off  InitialCurrent=0  Capacitance=1e-1  Setx0=off  InitialVoltage=0  Measurements=None
  Sine Wave2 : Sin  Commented=on  Amplitude=200  Bias=800  Frequency=3.14  Samples=2  SampleTime=1e-4
  Switch4 : Switch  Commented=on  Criteria=u2 > Threshold  Threshold=0.96  RndMeth=Ceiling  ZeroCross=off  SaturateOnIntegerOverflow=off
  Temperature : Constant  Value=25
  To Workspace : ToWorkspace  Commented=on  VariableName=IRsource  SaveFormat=Timeseries  SampleTime=-1
  To Workspace1 : ToWorkspace  VariableName=V_PV  SaveFormat=Timeseries  SampleTime=1e-4
      settings: Save2DSignal=2-D array (concatenate along first dimension)
  To Workspace2 : ToWorkspace  Commented=on  VariableName=x1  SaveFormat=Structure With Time  SampleTime=1
      settings: Decimation=2  Save2DSignal=2-D array (concatenate along first dimension)
  To Workspace3 : ToWorkspace  VariableName=I_PV  SaveFormat=Timeseries  SampleTime=1e-4
      settings: Save2DSignal=2-D array (concatenate along first dimension)
  To Workspace4 : ToWorkspace  VariableName=IR  SaveFormat=Timeseries  SampleTime=1e-4
      settings: Save2DSignal=2-D array (concatenate along first dimension)
  To Workspace5 : ToWorkspace  VariableName=P_Bat  SaveFormat=Timeseries  SampleTime=1e-4
      settings: Save2DSignal=2-D array (concatenate along first dimension)
  To Workspace6 : ToWorkspace  VariableName=DUTY  SaveFormat=Timeseries  SampleTime=1e-4
      settings: Save2DSignal=2-D array (concatenate along first dimension)
  To Workspace7 : ToWorkspace  VariableName=V_Bat  SaveFormat=Timeseries  SampleTime=1e-4
      settings: Save2DSignal=2-D array (concatenate along first dimension)
  Transport Delay : TransportDelay  Commented=on  DelayTime=10
  Type : Constant  Value=2  SampleTime=0
  extreme condition : Constant  Commented=on  Value=200
  output I and V : Scope  NumInputPorts=3
  zero : Constant  Commented=on  Value=0  SampleTime=0
  +Vo : PMIOPort  Side=Right
  -Vo : PMIOPort  Port=2  Side=Right
  tag scope: Vbb=global
  wires:
  [V_PV] -> Algorithm/3(V)
  [I_PV] -> Algorithm/2(I)
  Buck-Boost Converter/1(Outport) -> To Workspace7/1, Product/2, output I and V/2, [Vbb]  "voltage"
  Algorithm/1(duty) -> [duty]
  Type/1 -> Algorithm/1(Type)
  Bus Selector/2 -> [I_PV], Scope9/2, To Workspace3/1  "<I_PV>"
  Buck-Boost Converter/2(Outport1) -> Product/1, output I and V/1  "current"
  Bus Selector/1 -> To Workspace1/1, [V_PV], Scope9/1  "<V_PV>"
  PV Array1/1 -> Bus Selector/1
  [Vbb] -> Algorithm/5(Vbb)
  [Vtar] -> Algorithm/4(target)
  [duty] -> output I and V/3, To Workspace6/1  "duty cycle"
  [duty] -> Buck-Boost Converter/1(Inport)
  Algorithm/2(deltaw) -> Scope3/1
  Buck-Boost Converter/3(Outport2) -> [Vtar]
  Temperature/1 -> PV Array1/2
  Random Source/1 -> To Workspace/1, Transport Delay/1
  Transport Delay/1 -> Goto2/1, Scope1/1
  Repeating Sequence4/1 -> Switch4/2
  Random Source1/1 -> Switch4/1
  zero/1 -> Switch4/3
  extreme condition/1 -> Manual Switch/2
  Manual Switch/1 -> Goto6/1
  Switch4/1 -> Scope5/1, To Workspace2/1, Scope8/1, Manual Switch/1, Goto7/1
  Product/1 -> To Workspace5/1, Scope2/1
  IR2/1 -> Scope12/1, To Workspace4/1, PV Array1/1
  connections:
  PV Array1/RConn2 -- Buck-Boost Converter/LConn2 -- Series RLC Branch/RConn1
  PV Array1/RConn1 -- Series RLC Branch/LConn1 -- Diode1/LConn1
  Diode1/RConn1 -- Buck-Boost Converter/LConn1
  +Vo/RConn1 -- Buck-Boost Converter/RConn1
  -Vo/RConn1 -- Buck-Boost Converter/RConn2

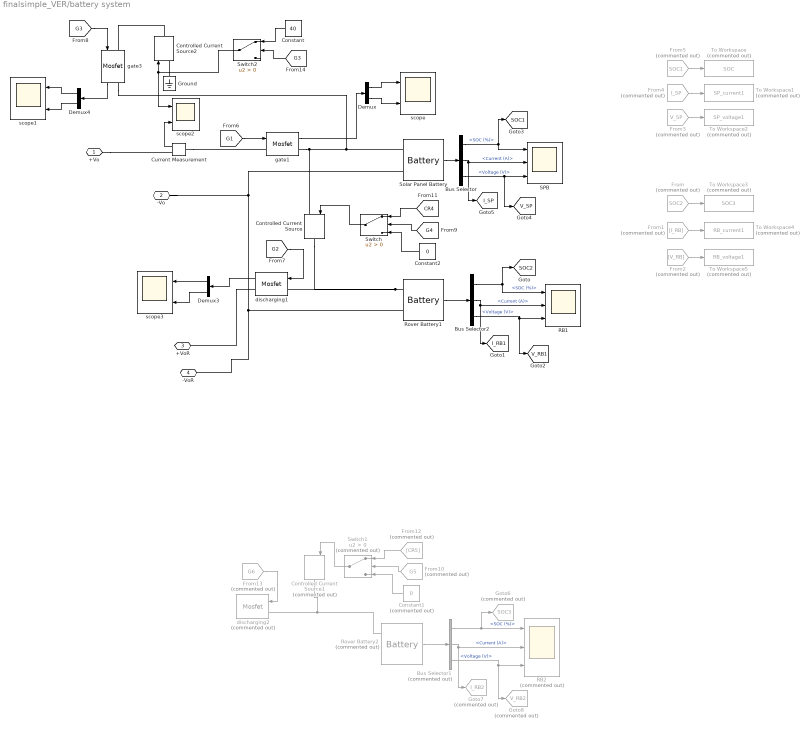
== system finalsimple_VER/battery system ==
  Bus Selector : BusSelector  OutputSignals=SOC (%),Current (A),Voltage (V)
  Bus Selector1 : BusSelector  Commented=on  OutputSignals=SOC (%),Current (A),Voltage (V)
  Bus Selector2 : BusSelector  OutputSignals=SOC (%),Current (A),Voltage (V)
  Constant : Constant  Value=40
  Constant1 : Constant  Commented=on  Value=0
  Constant2 : Constant  Value=0
  Controlled Current Source : spsControlledCurrentSourceLib/Controlled Current Source  Initialize=on  Source_Type=DC  Amplitude=150  Phase=0  Frequency=0  Measurements=Current
  Controlled Current Source1 : spsControlledCurrentSourceLib/Controlled Current Source  Commented=on  Initialize=on  Source_Type=DC  Amplitude=150  Phase=0  Frequency=0  Measurements=Current
  Controlled Current Source2 : spsControlledCurrentSourceLib/Controlled Current Source  Initialize=on  Source_Type=DC  Amplitude=100  Phase=0  Frequency=0  Measurements=Current
  Current Measurement : spsCurrentMeasurementLib/Current Measurement  PhasorSimulation=off  OutputType=Complex  PSBequivalent=0
  Demux : Demux  Outputs=2
  Demux3 : Demux  Outputs=2
  Demux4 : Demux  Outputs=2
  From : From  Commented=on  GotoTag=SOC2  TagVisibility=global
  From1 : From  Commented=on  GotoTag=I_RB  TagVisibility=global
  From10 : From  Commented=on  GotoTag=G5  TagVisibility=global
  From12 : From  Commented=on  GotoTag=CR5  TagVisibility=global
  From13 : From  Commented=on  GotoTag=G6  TagVisibility=global
  From2 : From  Commented=on  GotoTag=V_RB  TagVisibility=global
  From3 : From  Commented=on  GotoTag=V_SP  TagVisibility=global
  From4 : From  Commented=on  GotoTag=I_SP  TagVisibility=global
  From5 : From  Commented=on  GotoTag=SOC1  TagVisibility=global
  Goto6 : Goto  Commented=on  GotoTag=SOC3  TagVisibility=global
  Goto7 : Goto  Commented=on  GotoTag=I_RB2  TagVisibility=global
  Goto8 : Goto  Commented=on  GotoTag=V_RB2  TagVisibility=global
  Ground : spsGroundLib/Ground  LConnTagsString=a
  RB1 : Scope  NumInputPorts=3
  RB2 : Scope  Commented=on  NumInputPorts=3
  Rover Battery1 : spsBatteryLib/Battery  BatType=Lithium-Ion  ShowTempParam=off  ThermalPreset=no  ShowAgeParam=off  NomV=48  NomQ=50  SOC=50  Batt_Tr=3  PresetModel=off  MaxQ=50  MinV=36  FullV=52  Dis_rate=86.9565  R=0.0024  Normal_OP=48  expZone="[49.89      9.82609]"  current=[6.5 13 32.5]  Units=Time  Tci=25  NomT=20  T2=-30  MaxQ2=4.8  FullV2=7.1  Normal_OP2=5.655  expZone2="[6.58           1]"  Rca=0.6  ti=2000  Dp=0  Neq0=0  Tsim=1e6  Ta1=25  Qeol=5.4*0.9  Reol=0.013333*1.2  Char_age=[2.3478, 3]  Dis_age=[2.3478, 10]  N1=1500  N2=10500  N3=1000  N4=1400  Ta2=45  N5=950
  Rover Battery2 : spsBatteryLib/Battery  Commented=on  BatType=Lithium-Ion  ShowTempParam=off  ThermalPreset=no  ShowAgeParam=off  NomV=48  NomQ=50  SOC=50  Batt_Tr=3  PresetModel=off  MaxQ=50  MinV=36  FullV=52  Dis_rate=86.9565  R=0.0024  Normal_OP=48  expZone="[49.89      9.82609]"  current=[6.5 13 32.5]  Units=Time  Tci=25  NomT=20  T2=-30  MaxQ2=4.8  FullV2=7.1  Normal_OP2=5.655  expZone2="[6.58           1]"  Rca=0.6  ti=2000  Dp=0  Neq0=0  Tsim=1e6  Ta1=25  Qeol=5.4*0.9  Reol=0.013333*1.2  Char_age=[2.3478, 3]  Dis_age=[2.3478, 10]  N1=1500  N2=10500  N3=1000  N4=1400  Ta2=45  N5=950
  SPB : Scope  NumInputPorts=3
  Solar Panel Battery : spsBatteryLib/Battery  BatType=Lithium-Ion  ShowTempParam=off  ThermalPreset=no  ShowAgeParam=off  NomV=50  NomQ=100  SOC=50  Batt_Tr=3  PresetModel=off  MaxQ=100  MinV=36  FullV=55  Dis_rate=86.9565  R=0.0024  Normal_OP=98  expZone="[51.5     9.82609]"  current=[6.5 13 95]  Units=Time  Tci=25  NomT=20  T2=-30  MaxQ2=4.8  FullV2=7.1  Normal_OP2=5.655  expZone2="[6.58           1]"  Rca=0.6  ti=2000  Dp=0  Neq0=0  Tsim=1e6  Ta1=25  Qeol=5.4*0.9  Reol=0.013333*1.2  Char_age=[2.3478, 3]  Dis_age=[2.3478, 10]  N1=1500  N2=10500  N3=1000  N4=1400  Ta2=45  N5=950
  Switch : Switch  Criteria=u2 > Threshold  SaturateOnIntegerOverflow=off  InputSameDT=off
  Switch1 : Switch  Commented=on  Criteria=u2 > Threshold  SaturateOnIntegerOverflow=off  InputSameDT=off
  Switch2 : Switch  Criteria=u2 > Threshold  SaturateOnIntegerOverflow=off  InputSameDT=off
  To Workspace : ToWorkspace  Commented=on  VariableName=SOC  SampleTime=1
      settings: Decimation=2  Save2DSignal=2-D array (concatenate along first dimension)
  To Workspace1 : ToWorkspace  Commented=on  VariableName=SP_current1  SampleTime=1
      settings: Save2DSignal=2-D array (concatenate along first dimension)
  To Workspace2 : ToWorkspace  Commented=on  VariableName=SP_voltage1  SampleTime=1
      settings: Decimation=2  Save2DSignal=2-D array (concatenate along first dimension)
  To Workspace3 : ToWorkspace  Commented=on  VariableName=SOC3  SampleTime=1
      settings: Decimation=2  Save2DSignal=2-D array (concatenate along first dimension)
  To Workspace4 : ToWorkspace  Commented=on  VariableName=RB_current1  SampleTime=1
      settings: Decimation=2  Save2DSignal=2-D array (concatenate along first dimension)
  To Workspace5 : ToWorkspace  Commented=on  VariableName=RB_voltage1  SampleTime=1
      settings: Decimation=2  Save2DSignal=2-D array (concatenate along first dimension)
  discharging1 : spsMosfetLib/Mosfet  Ron=0.1  Lon=0  Rd=0.1  Vfd=80  IC=0  Rs=1e5  Cs=inf  Measurements=on
  discharging2 : spsMosfetLib/Mosfet  Commented=on  Ron=0.1  Lon=0  Rd=0.1  Vfd=80  IC=0  Rs=1e5  Cs=inf  Measurements=on
  gate1 : spsMosfetLib/Mosfet  Ron=0.1  Lon=0  Rd=0.1  Vfd=80  IC=0  Rs=1e5  Cs=inf  Measurements=on
  gate3 : spsMosfetLib/Mosfet  Ron=0.1  Lon=0  Rd=0.1  Vfd=80  IC=0  Rs=1e5  Cs=inf  Measurements=on
  scope{,1..3} (4 alike) : Scope  NumInputPorts=2
  +Vo : PMIOPort  Side=Left
  -Vo : PMIOPort  Port=2  Side=Left
  +VoR : PMIOPort  Port=3  Side=Left
  -VoR : PMIOPort  Port=4  Side=Left
  tag scope: I_RB1=global, I_SP=global, SOC1=global, SOC2=global, V_RB1=global, V_SP=global
  wires:
  From1/1 -> To Workspace4/1
  Bus Selector2/2 -> [I_RB1], RB1/2  "<Current (A)>"
  From/1 -> To Workspace3/1
  Bus Selector/1 -> SPB/1, [SOC1]  "<SOC (%)>"
  From5/1 -> To Workspace/1
  Rover Battery1/1 -> Bus Selector2/1
  Bus Selector/3 -> [V_SP], SPB/3  "<Voltage (V)>"
  From2/1 -> To Workspace5/1
  Bus Selector2/3 -> [V_RB1], RB1/3  "<Voltage (V)>"
  From3/1 -> To Workspace2/1
  From4/1 -> To Workspace1/1
  Bus Selector/2 -> [I_SP], SPB/2  "<Current (A)>"
  Solar Panel Battery/1 -> Bus Selector/1
  Bus Selector2/1 -> RB1/1, [SOC2]  "<SOC (%)>"
  [G1] -> gate1/1
  gate1/1 -> Demux/1
  Demux/1 -> scope/1
  Demux/2 -> scope/2
  discharging1/1 -> Demux3/1
  [G4] -> Switch/2
  Switch/1 -> Controlled Current Source/1
  [CR4] -> Switch/1
  Constant2/1 -> Switch/3
  [G2] -> discharging1/1
  Bus Selector1/1 -> Goto6/1, RB2/1  "<SOC (%)>"
  Bus Selector1/3 -> RB2/3, Goto8/1  "<Voltage (V)>"
  Rover Battery2/1 -> Bus Selector1/1
  Bus Selector1/2 -> RB2/2, Goto7/1  "<Current (A)>"
  Constant1/1 -> Switch1/3
  From12/1 -> Switch1/1
  From10/1 -> Switch1/2
  Switch1/1 -> Controlled Current Source1/1
  From13/1 -> discharging2/1
  Constant/1 -> Switch2/1
  Switch2/1 -> scope2/1, Controlled Current Source2/1
  gate3/1 -> Demux4/1
  [G3] -> gate3/1
  [G3] -> Switch2/2
  Demux4/1 -> scope1/1
  Demux4/2 -> scope1/2
  Current Measurement/1 -> scope2/2
  Demux3/1 -> scope3/1
  Demux3/2 -> scope3/2
  connections:
  Rover Battery1/LConn2 -- -VoR/RConn1 -- Solar Panel Battery/LConn2 -- -Vo/RConn1
  +Vo/RConn1 -- Current Measurement/RConn1
  Solar Panel Battery/LConn1 -- gate3/RConn1 -- gate1/RConn1 -- Controlled Current Source/LConn1
  Rover Battery1/LConn1 -- discharging1/LConn1 -- Controlled Current Source/RConn1
  discharging1/RConn1 -- +VoR/RConn1
  Rover Battery2/LConn1 -- Controlled Current Source1/RConn1 -- discharging2/LConn1
  Controlled Current Source2/RConn1 -- gate3/LConn1
  Ground/LConn1 -- Controlled Current Source2/LConn1
  Current Measurement/LConn1 -- gate1/LConn1
